simulink model "faultTolerantAircraft"  (R2023a)
settings: Solver=ode45  StartTime=0.0  StopTime=10  RelTol=1e-3  EnableMultiTasking=on
PreLoadFcn:
  | load faultTolerantAircraft
values from neighbouring files (symbols this model uses):
  Aac = [-0.00765 -0.0455 0.000222222222222 0 0 0 0.02405 -0.4784 0.00511111111111 0 0 0 ... (36 elements, 6x6)]    [faultTolerantAircraft.mat]
  alphaStep = 0    [faultTolerantAircraft.mat]
  Bac = [0.0108225 -0.2152575 0.0023 0 0 0 0.0053775 -0.038745 -0.04365 -0.0708525 -0.0946 -0.0839 ... (36 elements, 6x6)]    [faultTolerantAircraft.mat]
  betaStep = 0    [faultTolerantAircraft.mat]
  Cac = [0 0 0 -0.0344444444444 0 2.22222222222 0 0 0 0 0 0 ... (66 elements, 11x6)]    [faultTolerantAircraft.mat]
  Dac = [0 0 0 0 0 0 0 0 0 0 0 0 ... (66 elements, 11x6)]    [faultTolerantAircraft.mat]
  GustSpeed = 10    [FaultTolerantControl1.m]    (also in faultTolerantAircraft.mat)
  Ki = Ki.d    [FaultTolerantControl1.m]    (also in faultTolerantAircraft.mat = [1  0  0; 0  1  0; 0  0  1])
  Kx = Kx.d    [FaultTolerantControl1.m]    (also in faultTolerantAircraft.mat = [0 0 0 0 0 0 0 0 0 0 0 0 ... (18 elements, 3x6)])
  muStep = 0    [faultTolerantAircraft.mat]
  outage = [1 1 1 1 1]    [faultTolerantAircraft.mat]
libraries: simulink x2
settings Model: Creator=The MathWorks, Inc.  LastModifiedBy=The MathWorks, Inc.
settings SolverCC: AlgebraicLoopSolver=TrustRegion  MaxZcPerStep=1
settings DataIOCC: LimitDataPoints=on  SaveFormat=Array  ReturnWorkspaceOutputs=off
settings OptimizationCC: BlockReduction=off  BufferReuse=off  ExpressionDepthLimit=2147483647  LifeSpan=inf
settings DebuggingCC: AlgebraicLoopMsg=none  UnderspecifiedInitializationDetection=Classic  MergeDetectMultiDrivingBlocksExec=none  FcnCallInpInsideContextMsg=warning  StateNameClashWarn=warning  SFUnexpectedBacktrackingDiag=warning  SFNoUnconditionalDefaultTransitionDiag=warning  SFExecutionAtInitializationDiag=none  ArithmeticOperatorsInVariantConditions=warning
settings HardwareCC: ProdBitPerPointer=32  ProdBitPerSizeT=32  ProdBitPerPtrDiffT=32  ProdLargestAtomicFloat=None  ProdIntDivRoundTo=Undefined  ProdEndianess=Unspecified  ProdWordSize=32  ProdHWDeviceType=32-bit Generic
settings ModelReferenceCC: EnableRefExpFcnMdlSchedulingChecks=on  PropagateSignalLabelsOutOfModel=off
settings SFSimCC: SimUseLocalCustomCode=off  CustomCodeUndefinedFunction=UseInterfaceOnly
settings RTWCC: RTWUseLocalCustomCode=off  DLArmComputeVersion=19.05
settings CodeAppCC: StateflowObjectComments=on
settings GRTTargetCC: TargetLangStandard=C89/C90 (ANSI)
settings ConfigComp: CovMetricSettings=dw  CovSaveCumulativeToWorkspaceVar=on  CovSaveSingleToWorkspaceVar=on  CovExternalEMLEnable=off  CovSFcnEnable=off

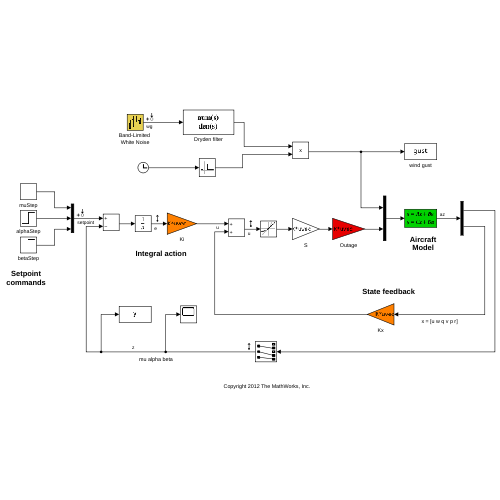
[thumbnail: Simulink's stored preview of the top-level diagram]
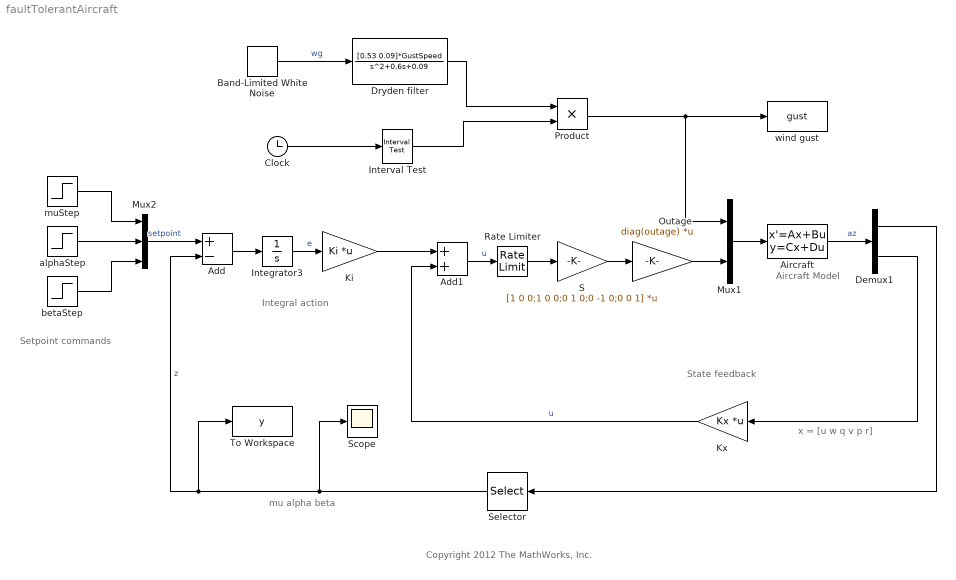
== system faultTolerantAircraft ==
  note: Copyright 2012 The MathWorks, Inc.
  note: Integral action
  note: x = [u w q v p r]
  note: mu alpha beta
  note: Setpoint
      | commands
  note: State feedback
  note: Aircraft
      | Model
  Add : Sum  Inputs=+-
  Add1 : Sum
  Aircraft : StateSpace  A=Aac  B=Bac  C=Cac  D=Dac  InitialCondition=0
  Band-Limited White Noise : simulink/Sources/Band-Limited White Noise  Cov=1  Ts=0.001  seed=[23341]
  Clock : Clock
  Demux1 : Demux  Outputs=2
  Dryden filter : TransferFcn  Numerator=[0.53 0.09]*GustSpeed  Denominator="[1  0.6  0.09]"
  Integrator3 : Integrator
  Interval Test : simulink/Logic and Bit Operations/Interval Test  IntervalClosedRight=on  uplimit=5  IntervalClosedLeft=on  lowlimit=0  OutDataTypeStr=boolean
  Ki : Gain  Gain=Ki  Multiplication=Matrix(K*u) (u vector)
  Kx : Gain  Gain=Kx  Multiplication=Matrix(K*u) (u vector)
  Mux1 : Mux  Inputs=2
  Mux2 : Mux  Inputs=3
  Outage : Gain  Gain=diag(outage)  Multiplication=Matrix(K*u) (u vector)
  Product : Product  RndMeth=Zero
  Rate Limiter : RateLimiter  RisingSlewLimit=60  FallingSlewLimit=-60  SampleTimeMode=inherited
  S : Gain  Gain=[1 0 0;1 0 0;0 1 0;0 -1 0;0 0 1]  Multiplication=Matrix(K*u) (u vector)
  Scope : Scope
  Selector : Selector  InputPortWidth=5  IndexOptions=Index vector (dialog)  Indices=[2 4 5]  OutputSizes=1
  To Workspace : ToWorkspace  VariableName=y  SaveFormat=Timeseries  SampleTime=-1
  alphaStep : Step  After=alphaStep  SampleTime=0
  betaStep : Step  After=betaStep  SampleTime=0
  muStep : Step  After=muStep  SampleTime=0
  wind gust : ToWorkspace  VariableName=gust  SaveFormat=Timeseries  SampleTime=-1
  wires:
  Clock/1 -> Interval Test/1
  Band-Limited White Noise/1 -> Dryden filter/1  "wg"
  Interval Test/1 -> Product/2
  Aircraft/1 -> Demux1/1  "az"
  Demux1/2 -> Kx/1
  Add/1 -> Integrator3/1
  Kx/1 -> Add1/2  "u"
  muStep/1 -> Mux2/1
  alphaStep/1 -> Mux2/2
  betaStep/1 -> Mux2/3
  Mux2/1 -> Add/1  "setpoint"
  S/1 -> Outage/1
  Outage/1 -> Mux1/2
  Integrator3/1 -> Ki/1  "e"
  Demux1/1 -> Selector/1
  Selector/1 -> Scope/1, To Workspace/1, Add/2  "z"
  Add1/1 -> Rate Limiter/1  "u"
  Rate Limiter/1 -> S/1
  Mux1/1 -> Aircraft/1
  Dryden filter/1 -> Product/1
  Product/1 -> wind gust/1, Mux1/1
  Ki/1 -> Add1/1
